simulink model "delay_force_pos_kalman"  (R2020b)
settings: Solver=ode45  StartTime=0.0  StopTime=10  FixedStep=Ts  MinStep=1e-5  RelTol=1e-5
undefined symbols (not defined in the file): A, A_int, b, B, Be, Bh_i, Bs, C, delayT, Dh, DiscIntNeverNeededParam, Discrete, Dm, Ds, Fc, Fip, Jh_i, Ke, Kh, Kh_i, Ks, Mm, Ms, R, Time, Ts, xe
libraries: ctrlSharedLib x2, cstblocks x1
settings Model: Creator=simon  LastModifiedBy=SimoneCremasco
settings SolverCC: AlgebraicLoopSolver=LineSearch

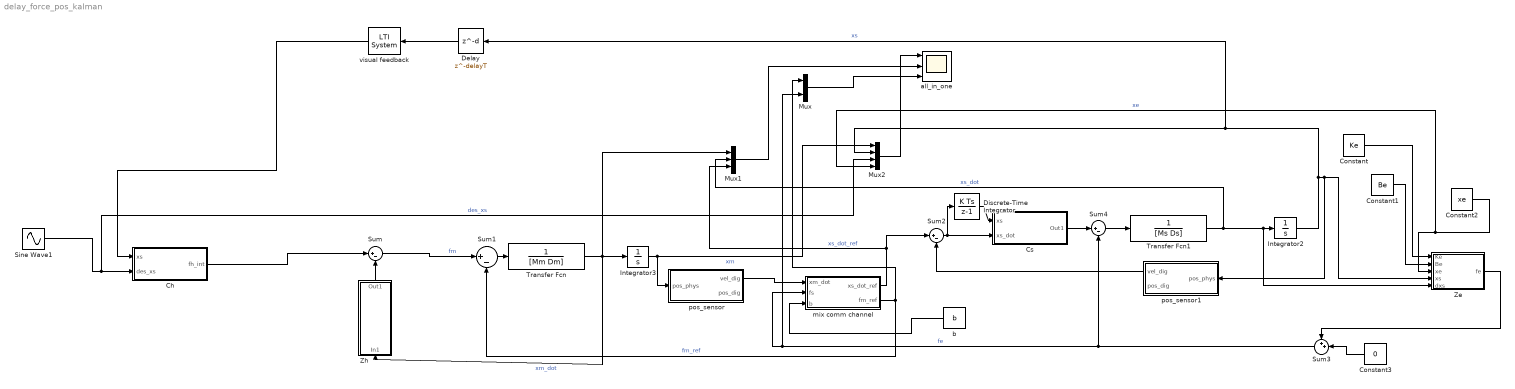
== system delay_force_pos_kalman ==
  Ch : Subsystem
  Constant : Constant  Value=Ke
  Constant1 : Constant  Value=Be
  Constant2 : Constant  Value=xe
  Constant3 : Constant  Value=0
  Cs : Subsystem
  Delay : Delay  DelayLength=delayT  SampleTime=Ts
  Discrete-Time Integrator : DiscreteIntegrator  SampleTime=-1  ICPrevOutput=DiscIntNeverNeededParam  ICPrevScaledInput=DiscIntNeverNeededParam
  Integrator2 : Integrator
  Integrator3 : Integrator
  Mux : Mux  Inputs=2
  Mux1 : Mux  Inputs=3
  Mux2 : Mux
  Sine Wave1 : Sin  Amplitude=A_int  Frequency=2*pi*Fc  SampleTime=0
  Sum{,1..2,4} (4 alike) : Sum  Inputs=|+-
  Sum3 : Sum  Inputs=++|
  Transfer Fcn : TransferFcn  Denominator=[Mm Dm]
  Transfer Fcn1 : TransferFcn  Denominator=[Ms Ds]
  Ze : MATLAB Function  TreatAsAtomicUnit=on
  Zh : Subsystem
  all_in_one : Scope  NumInputPorts=3
  b : Constant  Value=b
  mix comm channel : Subsystem
  pos_sensor : Subsystem
  pos_sensor1 : Subsystem
  visual feedback : cstblocks/LTI System  sys=1  IC=[]
  wires:
  Zh/1(Out1) -> Sum/2
  Sum1/1 -> Transfer Fcn/1
  Sum4/1 -> Transfer Fcn1/1
  Transfer Fcn1/1 -> Mux1/2, Integrator2/1, Ze/5(dxs)  "xs_dot"
  Ze/1(fe) -> Sum3/1
  Integrator2/1 -> Mux2/2, Delay/1, pos_sensor1/1(pos_phys), Ze/4(xs)  "xs"
  Constant2/1 -> Mux2/4, Ze/3(xe)  "xe"
  Constant1/1 -> Ze/2(Be)
  Constant/1 -> Ze/1(Ke)
  Sum/1 -> Sum1/1  "fm"
  Transfer Fcn/1 -> Mux1/1, Integrator3/1, Zh/1(In1)  "xm_dot"
  mix comm channel/2(fm_ref) -> Sum1/2, Mux/1  "fm_ref"
  mix comm channel/1(xs_dot_ref) -> Mux1/3, Sum2/1  "xs_dot_ref"
  Sum2/1 -> Discrete-Time Integrator/1, Cs/2(xs_dot)
  Discrete-Time Integrator/1 -> Cs/1(xs)
  Cs/1(Out1) -> Sum4/1
  Sum3/1 -> mix comm channel/2(fs), Mux/2, Sum4/2  "fe"
  Constant3/1 -> Sum3/2
  b/1 -> mix comm channel/3(b)
  Integrator3/1 -> Mux2/1, pos_sensor/1(pos_phys)  "xm"
  Sine Wave1/1 -> Mux2/3, Ch/2(des_xs)  "des_xs"
  Ch/1(fh_int) -> Sum/1
  visual feedback/1 -> Ch/1(xs)
  pos_sensor/1(vel_dig) -> mix comm channel/1(xm_dot)
  pos_sensor1/1(vel_dig) -> Sum2/2
  Delay/1 -> visual feedback/1
  Mux2/1 -> all_in_one/1
  Mux1/1 -> all_in_one/2
  Mux/1 -> all_in_one/3

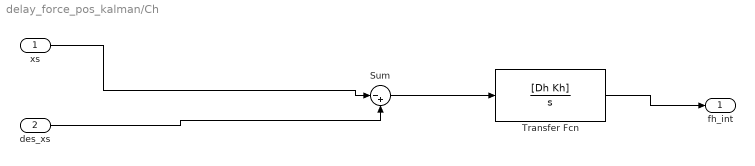
== system delay_force_pos_kalman/Ch ==
  xs : Inport
  des_xs : Inport  Port=2
  Sum : Sum  Inputs=|-+
  Transfer Fcn : TransferFcn  Numerator=[Dh Kh]  Denominator=[1 0]
  fh_int : Outport
  wires:
  xs/1 -> Sum/1
  des_xs/1 -> Sum/2
  Sum/1 -> Transfer Fcn/1
  Transfer Fcn/1 -> fh_int/1

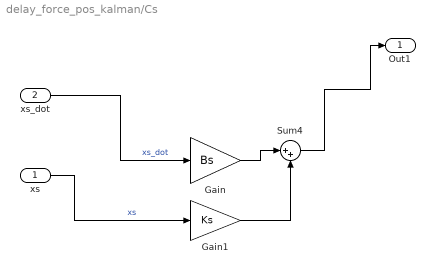
== system delay_force_pos_kalman/Cs ==
  xs : Inport
  xs_dot : Inport  Port=2
  Gain : Gain  Gain=Bs
  Gain1 : Gain  Gain=Ks
  Sum4 : Sum  Inputs=|++
  Out1 : Outport
  wires:
  Gain1/1 -> Sum4/2
  Sum4/1 -> Out1/1
  xs_dot/1 -> Gain/1  "xs_dot"
  Gain/1 -> Sum4/1
  xs/1 -> Gain1/1  "xs"

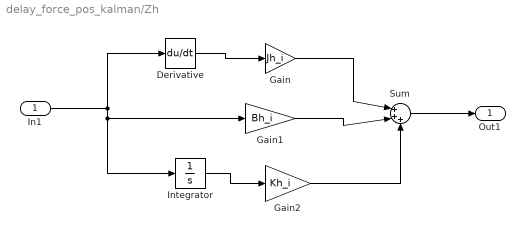
== system delay_force_pos_kalman/Zh ==
  In1 : Inport
  Derivative : Derivative
  Gain : Gain  Gain=Jh_i
  Gain1 : Gain  Gain=Bh_i
  Gain2 : Gain  Gain=Kh_i
  Integrator : Integrator
  Sum : Sum  Inputs=|+++
  Out1 : Outport
  wires:
  Derivative/1 -> Gain/1
  Integrator/1 -> Gain2/1
  In1/1 -> Integrator/1, Gain1/1, Derivative/1
  Gain/1 -> Sum/1
  Gain1/1 -> Sum/2
  Gain2/1 -> Sum/3
  Sum/1 -> Out1/1

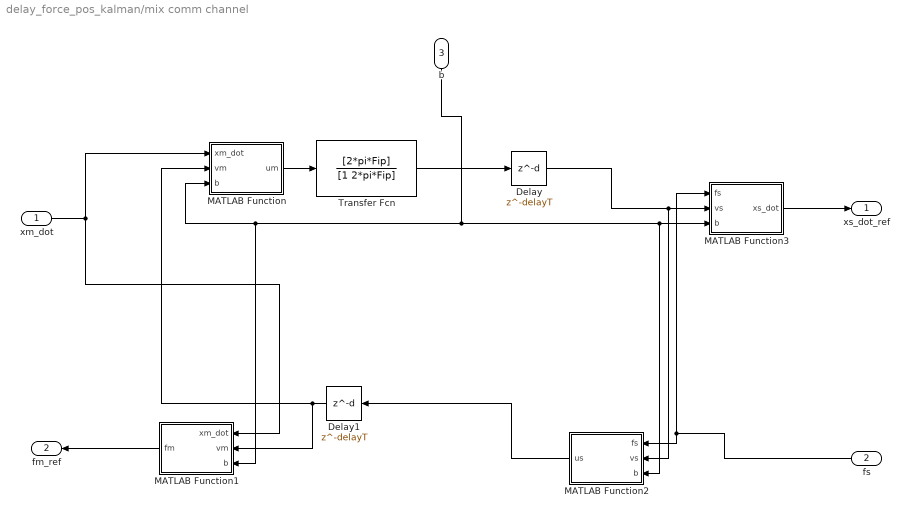
== system delay_force_pos_kalman/mix comm channel ==
  xm_dot : Inport
  fs : Inport  Port=2
  b : Inport  Port=3
  Delay : Delay  DelayLength=delayT  SampleTime=Ts
  Delay1 : Delay  DelayLength=delayT  SampleTime=Ts
  MATLAB Function : MATLAB Function  TreatAsAtomicUnit=on
  MATLAB Function1 : MATLAB Function  TreatAsAtomicUnit=on
  MATLAB Function2 : MATLAB Function  TreatAsAtomicUnit=on
  MATLAB Function3 : MATLAB Function  TreatAsAtomicUnit=on
  Transfer Fcn : TransferFcn  Numerator=[2*pi*Fip]  Denominator=[1 2*pi*Fip]
  xs_dot_ref : Outport
  fm_ref : Outport  Port=2
  wires:
  b/1 -> MATLAB Function1/3(b), MATLAB Function/3(b), MATLAB Function2/3(b), MATLAB Function3/3(b)
  xm_dot/1 -> MATLAB Function1/1(xm_dot), MATLAB Function/1(xm_dot)
  MATLAB Function1/1(fm) -> fm_ref/1
  fs/1 -> MATLAB Function3/1(fs), MATLAB Function2/1(fs)
  MATLAB Function3/1(xs_dot) -> xs_dot_ref/1
  MATLAB Function/1(um) -> Transfer Fcn/1
  Delay/1 -> MATLAB Function2/2(vs), MATLAB Function3/2(vs)
  Delay1/1 -> MATLAB Function/2(vm), MATLAB Function1/2(vm)
  Transfer Fcn/1 -> Delay/1
  MATLAB Function2/1(us) -> Delay1/1

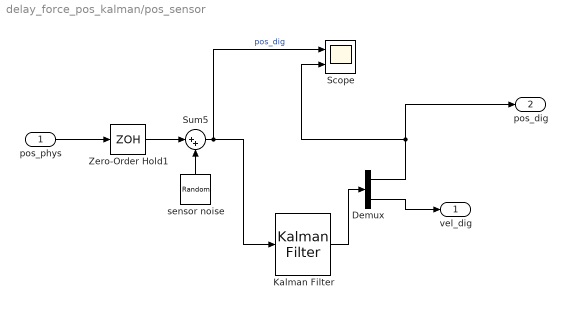
== system delay_force_pos_kalman/pos_sensor ==
  pos_phys : Inport
  Demux : Demux  Outputs=2
  Kalman Filter : ctrlSharedLib/Kalman Filter  TimeDomain=Discrete-Time  UseCurrentEstimator=on  ModelSource=Individual A, B, C, D matrices  ModelSourceVariable=ss(0.95,1,1,0,1)  A=A  B=B  C=C  D=0  NumberOfStates=2  NumberOfInputs=1  NumberOfOutputs=1  InitialEstimateSource=Dialog  X0=0  P0=10  UseK=off  UseGH=off  NumberOfProcessNoiseInputs=1  G=1  TimeInvariantG=on  H=0  TimeInvariantH=on  Q=Q_m  TimeInvariantQ=on  R=R  TimeInvariantR=on  N=0  TimeInvariantN=on  AddInputPort=off  AddEnablePort=off  OutputEstimatedY=off  OutputP=off  Ts=Ts
  Scope : Scope  NumInputPorts=2
  Sum5 : Sum  Inputs=|++
  Zero-Order Hold1 : ZeroOrderHold  SampleTime=Ts
  sensor noise : RandomNumber  Variance=0.00000001  SampleTime=Ts
  vel_dig : Outport
  pos_dig : Outport  Port=2
  wires:
  Zero-Order Hold1/1 -> Sum5/1
  sensor noise/1 -> Sum5/2
  pos_phys/1 -> Zero-Order Hold1/1
  Sum5/1 -> Scope/1, Kalman Filter/1  "pos_dig"
  Kalman Filter/1 -> Demux/1
  Demux/1 -> pos_dig/1, Scope/2
  Demux/2 -> vel_dig/1

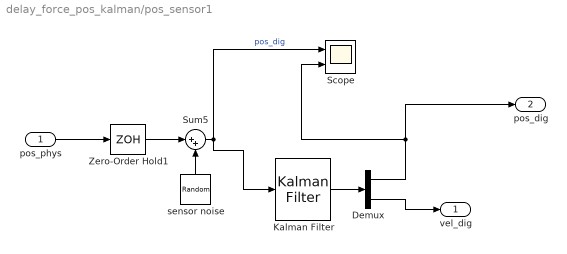
== system delay_force_pos_kalman/pos_sensor1 ==
  pos_phys : Inport
  Demux : Demux  Outputs=2
  Kalman Filter : ctrlSharedLib/Kalman Filter  TimeDomain=Discrete-Time  UseCurrentEstimator=on  ModelSource=Individual A, B, C, D matrices  ModelSourceVariable=ss(0.95,1,1,0,1)  A=A  B=B  C=C  D=0  NumberOfStates=2  NumberOfInputs=1  NumberOfOutputs=1  InitialEstimateSource=Dialog  X0=0  P0=10  UseK=off  UseGH=off  NumberOfProcessNoiseInputs=1  G=1  TimeInvariantG=on  H=0  TimeInvariantH=on  Q=Q_s  TimeInvariantQ=on  R=R  TimeInvariantR=on  N=0  TimeInvariantN=on  AddInputPort=off  AddEnablePort=off  OutputEstimatedY=off  OutputP=off  Ts=Ts
  Scope : Scope  NumInputPorts=2
  Sum5 : Sum  Inputs=|++
  Zero-Order Hold1 : ZeroOrderHold  SampleTime=Ts
  sensor noise : RandomNumber  Variance=0.00000001  SampleTime=Ts
  vel_dig : Outport
  pos_dig : Outport  Port=2
  wires:
  Zero-Order Hold1/1 -> Sum5/1
  sensor noise/1 -> Sum5/2
  pos_phys/1 -> Zero-Order Hold1/1
  Sum5/1 -> Scope/1, Kalman Filter/1  "pos_dig"
  Kalman Filter/1 -> Demux/1
  Demux/1 -> pos_dig/1, Scope/2
  Demux/2 -> vel_dig/1

== matlab function delay_force_pos_kalman/Ze ==
  data: Ke input; fe output; Be input; xe input; xs input; dxs input
function fe = env(Ke, Be, xe, xs, dxs)
    if xs > xe
        fe = Ke*(xs-xe)+Be*max(dxs, 0);
    else
        fe = 0;
    end

== matlab function delay_force_pos_kalman/mix comm channel/MATLAB Function ==
  data: xm_dot input; um output; vm input; b input
function um = fcn(xm_dot, vm, b)

um = sqrt(2*b)*xm_dot+vm;

== matlab function delay_force_pos_kalman/mix comm channel/MATLAB Function1 ==
  data: xm_dot input; fm output; vm input; b input
function fm = fcn(xm_dot, vm, b)

fm = b*xm_dot+sqrt(2*b)*vm;

== matlab function delay_force_pos_kalman/mix comm channel/MATLAB Function2 ==
  data: fs input; us output; vs input; b input
function us = fcn(fs, vs, b)

us = sqrt(2/b)*fs-vs;

== matlab function delay_force_pos_kalman/mix comm channel/MATLAB Function3 ==
  data: fs input; xs_dot output; vs input; b input
function xs_dot = fcn(fs, vs, b)

xs_dot = -1/b*(fs-sqrt(2*b)*vs);
